simulink model "test_positioning_simulink"  (R2015a)
settings: Solver=ode45  StartTime=0.0  StopTime=10.0  RelTol=1e-3
values from neighbouring files (symbols this model uses):
  field_x = abs(CR1(1) - CR2(1) + CR4(1) - CR3(1))/2    [CalibrateField.m]    (also in Config.mat = 11.1837954032)
  field_y = abs(CR4(2) - CR1(2) + CR3(2) - CR2(2))/2    [CalibrateField.m]    (also in Config.mat = 7.36656071895)
settings Model: Creator=tzwijger  LastModifiedBy=tzwijger

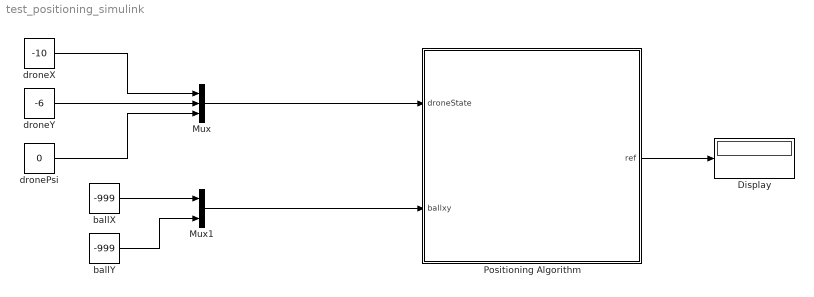
== system test_positioning_simulink ==
  Display : Display
  Mux : Mux  Inputs=3
  Mux1 : Mux  Inputs=2
  Positioning Algorithm : Subsystem
  ballX : Constant  Value=-999
  ballY : Constant  Value=-999
  dronePsi : Constant  Value=0
  droneX : Constant  Value=-10
  droneY : Constant  Value=-6
  wires:
  Mux/1 -> Positioning Algorithm/1(droneState)
  droneX/1 -> Mux/1
  droneY/1 -> Mux/2
  dronePsi/1 -> Mux/3
  Positioning Algorithm/1(ref) -> Display/1
  Mux1/1 -> Positioning Algorithm/2(ballxy)
  ballX/1 -> Mux1/1
  ballY/1 -> Mux1/2

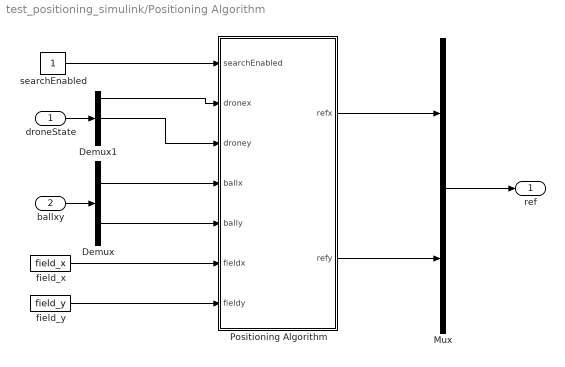
== system test_positioning_simulink/Positioning Algorithm ==
  droneState : Inport
  ballxy : Inport  Port=2
  Demux : Demux  Outputs=2
  Demux1 : Demux  Outputs=3
  Mux : Mux  Inputs=2
  Positioning Algorithm : MATLAB Function  TreatAsAtomicUnit=on
  field_x : Constant  Value=field_x
  field_y : Constant  Value=field_y
  searchEnabled : Constant
  ref : Outport
  wires:
  Demux/2 -> Positioning Algorithm/5(bally)
  Demux/1 -> Positioning Algorithm/4(ballx)
  Positioning Algorithm/1(refx) -> Mux/1
  Positioning Algorithm/2(refy) -> Mux/2
  Mux/1 -> ref/1
  field_x/1 -> Positioning Algorithm/6(fieldx)
  field_y/1 -> Positioning Algorithm/7(fieldy)
  droneState/1 -> Demux1/1
  ballxy/1 -> Demux/1
  Demux1/2 -> Positioning Algorithm/3(droney)
  searchEnabled/1 -> Positioning Algorithm/1(searchEnabled)
  Demux1/1 -> Positioning Algorithm/2(dronex)

== matlab function test_positioning_simulink/Positioning Algorithm/Positioning Algorithm ==
  data: searchEnabled input; dronex input; droney input; ballx input; refx output; bally input; refy output; fieldx input; fieldy input
function [refx,refy] = positionDrone(searchEnabled,dronex,droney,ballx,bally,fieldx,fieldy)
% ball position [-999 -999] -> No Ball Position Known
    persistent searchArray count step
    if isempty(searchArray)
       count = 1;
       i = 1;
       step = 1;
       searchArray = zeros(100,2);% Size HAS to be predetermined (...Simulink...)
       for y = -0.5*fieldy:step:0.5*fieldy
          searchArray(i,:) =  [-0.5*fieldx,y];
          searchArray(i+1,:) =  [0.5*fieldx,y];
          i = i + 2;
       end
    end
    refx = 0;
    refy = 0;

    if ballx ~= -999 && bally ~= -999
        % Ball Position is known
        if abs(ballx) < 0.5*fieldx && abs(bally) < 0.5*fieldy
            % Ball is in field
            refx = ballx; 
            refy = bally;
        else
            % Ball is out of field
            % Go as close as possible without leaving the field
            refx = sign(ballx)*min(abs(ballx),0.5*fieldx);
            refy = sign(bally)*min(abs(bally),0.5*fieldy);       
        end
        % Reset count if search was enabled
        if count ~= 1
            count = 1;
        end
    elseif searchEnabled
        % Ball position is not known, search sequence initiated
        if (abs(dronex) - searchArray(count,1) < 0.25 ||...
            abs(droney) - searchArray(count,2) < 0.25)
            if count < 2*floor(fieldy/step)
                count = count + 1;
            else
                count = 1;
            end
        end
        refx = searchArray(count,1);
        refy = searchArray(count,2);
    else
        % Search disabled, hover over origin
        refx = 0;
        refy = 0;
    end
